simulink model "StateSpaceResults"  (R2023a)
settings: Solver=VariableStepAuto  StartTime=0.0  StopTime=10  RelTol=1e-3
undefined symbols (not defined in the file or in its folder): den1, den2, num1, num2
settings Model: Creator=minim  LastModifiedBy=minim

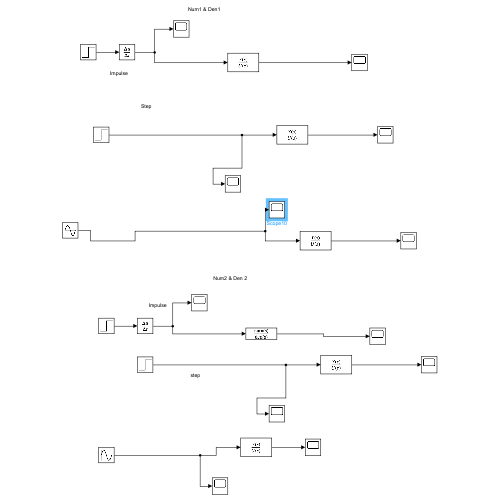
[thumbnail: Simulink's stored preview of the top-level diagram]
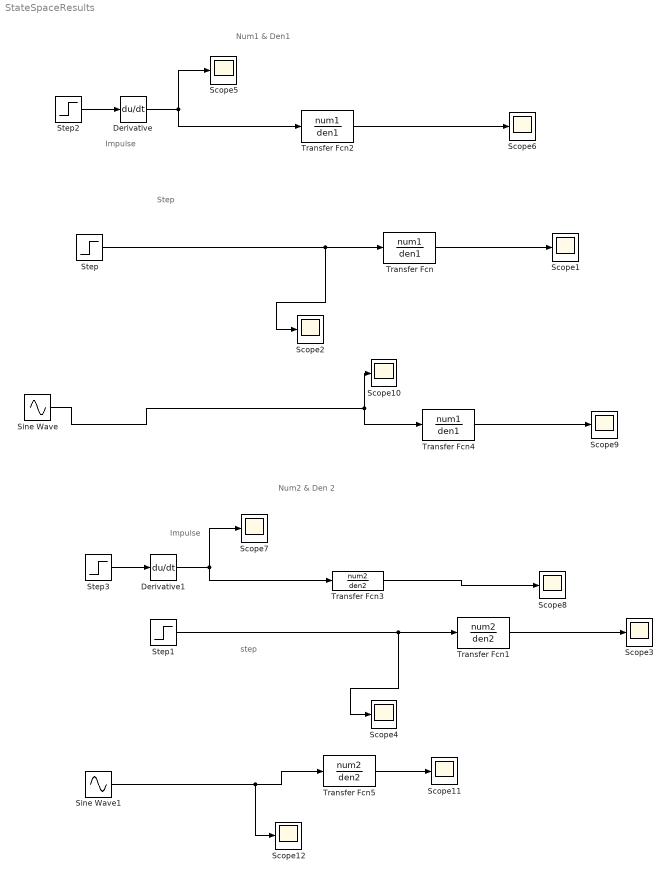
== system StateSpaceResults ==
  note: Impulse
  note: Num2 & Den 2
  note: Num1 & Den1
  note: Step
  note: step
  note: Impulse
  Derivative : Derivative  CoefficientInTFapproximation=0
  Derivative1 : Derivative  CoefficientInTFapproximation=0
  Scope{1..12} (12 alike) : Scope
  Sine Wave : Sin  SampleTime=0  VectorParams1D=off
  Sine Wave1 : Sin  SampleTime=0  VectorParams1D=off
  Step : Step  After=0.1  SampleTime=0
  Step1 : Step  After=0.1  SampleTime=0
  Step2 : Step  SampleTime=0
  Step3 : Step  SampleTime=0
  Transfer Fcn : TransferFcn  Numerator=num1  Denominator=den1
  Transfer Fcn1 : TransferFcn  Numerator=num2  Denominator=den2
  Transfer Fcn2 : TransferFcn  Numerator=num1  Denominator=den1
  Transfer Fcn3 : TransferFcn  Numerator=num2  Denominator=den2
  Transfer Fcn4 : TransferFcn  Numerator=num1  Denominator=den1
  Transfer Fcn5 : TransferFcn  Numerator=num2  Denominator=den2
  wires:
  Step2/1 -> Derivative/1
  Derivative/1 -> Scope5/1, Transfer Fcn2/1
  Transfer Fcn2/1 -> Scope6/1
  Step/1 -> Transfer Fcn/1, Scope2/1
  Step3/1 -> Derivative1/1
  Transfer Fcn/1 -> Scope1/1
  Transfer Fcn1/1 -> Scope3/1
  Step1/1 -> Scope4/1, Transfer Fcn1/1
  Derivative1/1 -> Scope7/1, Transfer Fcn3/1
  Transfer Fcn3/1 -> Scope8/1
  Sine Wave/1 -> Transfer Fcn4/1, Scope10/1
  Transfer Fcn4/1 -> Scope9/1
  Transfer Fcn5/1 -> Scope11/1
  Sine Wave1/1 -> Transfer Fcn5/1, Scope12/1
